simulink model "MissileGuidanceMainBlockTrail1"  (R2015a)
settings: Solver=ode45  StartTime=0.0  StopTime=100  RelTol=1e-5
libraries: simulink x1
settings Model: CovSFcnEnable=off  Creator=Mostafa  LastModifiedBy=Rushdi
settings DebuggingCC: SolverPrmCheckMsg=warning

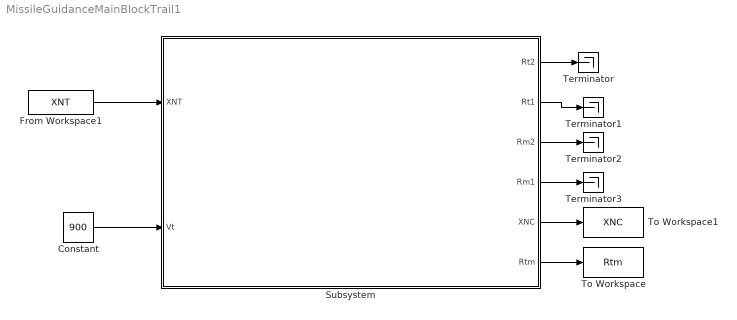
== system MissileGuidanceMainBlockTrail1 ==
  Constant : Constant  Value=900
  From Workspace1 : FromWorkspace  VariableName=XNT  SampleTime=0
  Subsystem : Subsystem
  Terminator{,1..3} (4 alike) : Terminator
  To Workspace : ToWorkspace  VariableName=Rtm  SampleTime=-1
  To Workspace1 : ToWorkspace  VariableName=XNC  SampleTime=-1
  wires:
  Constant/1 -> Subsystem/2(Vt)
  Subsystem/1(Rt2) -> Terminator/1
  Subsystem/2(Rt1) -> Terminator1/1
  Subsystem/3(Rm2) -> Terminator2/1
  Subsystem/4(Rm1) -> Terminator3/1
  Subsystem/5(XNC) -> To Workspace1/1
  Subsystem/6(Rtm) -> To Workspace/1
  From Workspace1/1 -> Subsystem/1(XNT)

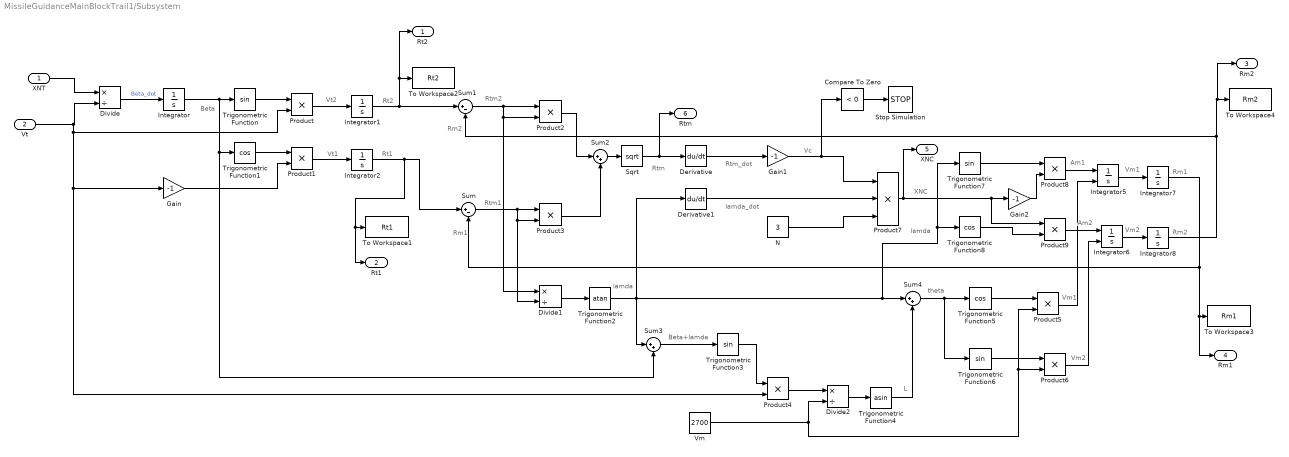
== system MissileGuidanceMainBlockTrail1/Subsystem ==
  note: Rm2
  note: Rm1
  note: Vm1
  note: Vm2
  note: Am2
  note: Am1
  note: lamda
  note: XNC
  note: lamda_dot
  note: Vc
  note: Rtm_dot
  note: Rtm
  note: Vm2
  note: Vm1
  note: theta
  note: L
  note: Beta+lamda
  note: lamda
  note: Rtm2
  note: Rm2
  note: Rtm1
  note: Rm1
  note: Rt1
  note: Rt2
  note: Vt2
  note: Vt1
  note: Beta
  XNT : Inport
  Vt : Inport  Port=2
  Compare To Zero : simulink/Logic and Bit Operations/Compare To Zero  relop=<  OutDataTypeStr=boolean  ZeroCross=off
  Derivative : Derivative
  Derivative1 : Derivative
  Divide : Product  Inputs=*/
  Divide1 : Product  Inputs=*/
  Divide2 : Product  Inputs=*/
  Gain : Gain  Gain=-1
  Gain1 : Gain  Gain=-1
  Gain2 : Gain  Gain=-1
  Integrator : Integrator
  Integrator1 : Integrator  InitialCondition=10000
  Integrator2 : Integrator  InitialCondition=12000
  Integrator5 : Integrator  InitialConditionSource=external
  Integrator6 : Integrator  InitialConditionSource=external
  Integrator7 : Integrator
  Integrator8 : Integrator  InitialCondition=9000
  N : Constant  Value=3
  Product{,1..6,8..9} (9 alike) : Product
  Product7 : Product  Inputs=3
  Sqrt : Sqrt  SaturateOnIntegerOverflow=on
  Stop Simulation : Stop
  Sum : Sum  Inputs=|+-
  Sum1 : Sum  Inputs=|+-
  Sum2 : Sum  Inputs=|++
  Sum3 : Sum  Inputs=|++
  Sum4 : Sum  Inputs=|++
  To Workspace1 : ToWorkspace  VariableName=Rt1  SampleTime=-1
  To Workspace2 : ToWorkspace  VariableName=Rt2  SampleTime=-1
  To Workspace3 : ToWorkspace  VariableName=Rm1  SampleTime=-1
  To Workspace4 : ToWorkspace  VariableName=Rm2  SampleTime=-1
  Trigonometric Function{,3,6..7} (4 alike) : Trigonometry
  Trigonometric Function1 : Trigonometry  Operator=cos
  Trigonometric Function2 : Trigonometry  Operator=atan
  Trigonometric Function4 : Trigonometry  Operator=asin
  Trigonometric Function5 : Trigonometry  Operator=cos
  Trigonometric Function8 : Trigonometry  Operator=cos
  Vm : Constant  Value=2700
  Rt2 : Outport
  Rt1 : Outport  Port=2
  Rm2 : Outport  Port=3
  Rm1 : Outport  Port=4
  XNC : Outport  Port=5
  Rtm : Outport  Port=6
  wires:
  XNT/1 -> Divide/1
  Vt/1 -> Gain/1, Product4/2, Product/2, Divide/2
  Divide/1 -> Integrator/1  "Beta_dot"
  Integrator/1 -> Sum3/2, Trigonometric Function1/1, Trigonometric Function/1
  Trigonometric Function/1 -> Product/1
  Gain/1 -> Product1/2
  Trigonometric Function1/1 -> Product1/1
  Product1/1 -> Integrator2/1
  Product/1 -> Integrator1/1
  Integrator1/1 -> Rt2/1, To Workspace2/1, Sum1/1
  Integrator2/1 -> Rt1/1, To Workspace1/1, Sum/1
  Sum1/1 -> Product2/2, Divide1/1, Product2/1
  Sum/1 -> Divide1/2, Product3/2, Product3/1
  Product2/1 -> Sum2/1
  Product3/1 -> Sum2/2
  Sum2/1 -> Sqrt/1
  Divide1/1 -> Trigonometric Function2/1
  Trigonometric Function2/1 -> Derivative1/1, Sum3/1, Trigonometric Function7/1, Trigonometric Function8/1, Sum4/1
  Sum3/1 -> Trigonometric Function3/1
  Trigonometric Function3/1 -> Product4/1
  Product4/1 -> Divide2/1
  Vm/1 -> Divide2/2, Product5/2, Product6/2
  Divide2/1 -> Trigonometric Function4/1
  Trigonometric Function4/1 -> Sum4/2
  Sum4/1 -> Trigonometric Function6/1, Trigonometric Function5/1
  Trigonometric Function5/1 -> Product5/1
  Trigonometric Function6/1 -> Product6/1
  Sqrt/1 -> Rtm/1, Derivative/1
  Derivative/1 -> Gain1/1
  Gain1/1 -> Compare To Zero/1, Product7/1
  Derivative1/1 -> Product7/2
  N/1 -> Product7/3
  Product7/1 -> XNC/1, Product9/1, Gain2/1
  Trigonometric Function8/1 -> Product9/2
  Gain2/1 -> Product8/2
  Trigonometric Function7/1 -> Product8/1
  Product8/1 -> Integrator5/1
  Product9/1 -> Integrator6/1
  Integrator6/1 -> Integrator8/1
  Integrator5/1 -> Integrator7/1
  Compare To Zero/1 -> Stop Simulation/1
  Integrator8/1 -> Rm2/1, To Workspace4/1, Sum1/2
  Integrator7/1 -> Rm1/1, To Workspace3/1, Sum/2
  Product6/1 -> Integrator6/2
  Product5/1 -> Integrator5/2
